simulink model "untitled1"  (R2020b)
settings: Solver=VariableStepAuto  StartTime=0.0  StopTime=10.0  RelTol=1e-3
settings Model: Creator=Javad  LastModifiedBy=Javad

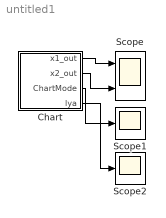
== system untitled1 ==
  Chart : Stateflow chart  TreatAsAtomicUnit=on
  Scope : Scope  NumInputPorts=2
  Scope1 : Scope
  Scope2 : Scope
  wires:
  Chart/2(x2_out) -> Scope/2
  Chart/1(x1_out) -> Scope/1
  Chart/3(ChartMode) -> Scope1/1
  Chart/4(lya) -> Scope2/1

== stateflow chart untitled1/Chart ==
  settings: updateMethod=CONTINUOUS
  state Q1
    du:
    x1_dot=10*x2;
    x2_dot=0;
    x1_out=x1;
    x2_out=x2;
    lya=x1^2+x2^2;
  state Q2
    du:
    x1_dot=1.5*x1+2*x2;
    x2_dot=-2*x1-0.5*x2 ;
    x1_out=x1;
    x2_out=x2;
    lya=x1^2+x2^2;
  (default) -> Q1 : {x1=-5;x2=2;}
  Q1 -> Q2 : [((x1<0 || x2<-0.25*x1 || x2>0.5*x1) && (x1>=0 || x2<0.5*x1 || x2>-0.25*x1)) ]
      | {x1=x1;x2=x2;}
  Q2 -> Q1 : [((x1>=0 && x2>=-0.25*x1 && x2<=0.5*x1) || (x1<0 && x2>=0.5*x1 && x2<=-0.25*x1))]
      | {x1=x1;x2=x2;}
  data: x1_out output; x2_out output; x2 local; x1 local; ChartMode output Enum: ChartModeType; lya output
  data x2 settings: updateMethod=SF_CONTINUOUS_TIME_DATA
  data x1 settings: updateMethod=SF_CONTINUOUS_TIME_DATA
